simulink model "admire_fcs_lin"  (Simulink 3.00)
settings: Solver=ode4  SolverMode=SingleTasking  StartTime=0.0  StopTime=60  FixedStep=0.008  RelTol=1e-3  AbsTol=1e-6
values from neighbouring files (symbols this model uses):
  x0 = [ max(eyp,zeros(n,1));max(-eyp,zeros(n,1));zeros(2*m,1)]    [LPwrap.m]
undefined symbols (not defined in the file or in its folder): Alt, dalt_err, dMach_err, Mach, u0fcs, y0bare
libraries: simulink3 x22, simulink_extras x8
settings Model: TimeSaveName=tout_split  SaveState=on  StateSaveName=xout_split  OutputSaveName=yout_split  RTWOptions="-aLogVarNameModifier=\"rt_\" -aExtMode=0 -aRollThreshold=5 -aShowEliminatedStatements=1 -aRTWVerbose=1 -aInlineInvariantSignals=1 -aLocalBlockOutputs=1 -aInlineParameters=0"  RTWTemplateMakefile=grt_adm5p3.tmf  LastModifiedBy=lkh  ModifiedComment=nnt -- Mon Jun 05 13:08:11 2000 -- Version 3.42
settings Model: ModifiedHistory=|
  | hkg-- Wed Apr 18 2001: Bug fix: dMach_err and dalt_err are now added to Mach and Alt
  | hkg-- Fri Apr 06 2001: Released with Admire version 3.4d
  | nnt -- Mon Jun 05 13:08:11 2000 -- Version 3.42
  | nnt -- Mon Jun 05 11:01:33 2000 -- Version 3.41
  | nnt -- Mon Jun 05 10:57:40 2000 -- Version 3.40
  | nnt -- Mon Jun 05 10:56:46 2000 -- Version 3.39
  | hkg -- Thu Apr 13 16:38:30 2000 -- Version 3.38
  | Bug fix: all rate limiters were set with the canard parameters, now they get individual settings..
  | hkg -- Thu Apr 13 10:24:31 2000 -- Version 3.37
  | Inserted 3.0 version number in Level 1, changed month to April.
  | hkg -- Tue Apr 11 10:36:55 2000 -- Version 3.36
  | dtz re-connected
  | hkg -- Tue Apr 11 10:28:52 2000 -- Version 3.35
  | Changed the roll force saturation to +-80 N
  | hkg -- Tue Apr 11 09:23:02 2000 -- Version 3.34
  | All signal generators on Level 1 are now set to sine wave
  | hkg -- Mon Apr 10 15:03:16 2000 -- Version 3.33
  | New names for the RL_choice blocks
  | fosimadmin -- Mon Apr 10 13:44:14 2000 -- Version 3.32
  | Hkg actually. Nothing special
  | hkg -- Fri Apr 07 14:32:16 2000 -- Version 3.31
  | A few corrections to the names
  | hkg -- Fri Apr 07 14:16:55 2000 -- Version 3.30
  | Added unique names inside Saab and DASA rate limiters for left elevons, rudder and
  | leading-edge flaps.
  | hkg -- Fri Apr 07 14:04:35 2000 -- Version 3.29
  | Added unique names inside SAAB and DASA rate limiters for canard and right outer and
  | inner elevons.
  | hkg -- Thu Apr 06 17:23:24 2000 -- Version 3.28
  | Inserted unique names for rate limiters and multiport switches in the rate limiter selection blocks.
  | hkg -- Thu Apr 06 16:09:22 2000 -- Version 3.27
  | Disconnected dtz again. Chosen grt_adm5p3.tmf as template makefile. Code generation seems to work.
  | hyd -- Tue Mar 28 15:20:39 2000 -- Version 3.26
  | hyd -- Tue Mar 28 14:28:32 2000 -- Version 3.25
  | hyd -- Tue Mar 28 11:30:24 2000 -- Version 3.24
  | hyd -- Mon Mar 27 15:22:27 2000 -- Version 3.23
  | hyd -- Mon Mar 27 13:42:12 2000 -- Version 3.22
  | hyd -- Mon Mar 27 10:51:54 2000 -- Version 3.21
  | hyd -- Fri Mar 24 13:18:05 2000 -- Version 3.20
  | hyd -- Fri Mar 24 12:50:02 2000 -- Version 3.19
  | hyd -- Fri Mar 24 11:54:23 2000 -- Version 3.18
  | hyd -- Thu Mar 23 15:20:42 2000 -- Version 3.17
  | hyd -- Thu Mar 23 15:17:54 2000 -- Version 3.16
  | hyd -- Wed Mar 22 09:38:49 2000 -- Version 3.15
  | hyd -- Tue Mar 21 14:06:08 2000 -- Version 3.14
  | hyd -- Mon Mar 20 14:42:54 2000 -- Version 3.13
  | hyd -- Wed Mar 15 13:37:48 2000 -- Version 3.12
  | hyd -- Wed Mar 15 12:35:54 2000 -- Version 3.11
  | jnr -- Tue Mar 14 16:36:26 2000 -- Version 3.10
  | jnr -- Tue Mar 14 14:13:39 2000 -- Version 3.9
  | jnr -- Tue Mar 14 14:13:23 2000 -- Version 3.8
  | jnr -- Tue Mar 14 10:09:15 2000 -- Version 3.7
  | jnr -- Tue Mar 14 09:37:34 2000 -- Version 3.6
  | jnr -- Tue Mar 14 09:30:20 2000 -- Version 3.5
  | Add:
  | *proper stick gradients.
  | *correct gains for nz-control according to Åke Hydén.
  | *what transition region between q-control and nz-control is proper??
  | fll -- Fri Mar 03 09:53:48 2000 -- Version 3.4
  | changed name of "dtx" to "dty" (horizontal nozzle deflection)
  | fll -- Thu Mar 02 12:51:23 2000 -- Version 3.3
  | Reducesed the number of integrators to one in the longitudinal controller.
  | fll -- Thu Mar 02 12:30:52 2000 -- Version 3.2
  | Moved the blending function in the Nz and q controller.
  | fll -- Thu Mar 02 10:50:25 2000 -- Version 3.1
  | Changed input blocks to "Signal generator"
  | fll -- Thu Mar 02 10:50:25 2000 -- Version 3.0
  | Version 3.0 is modified according to comments from users

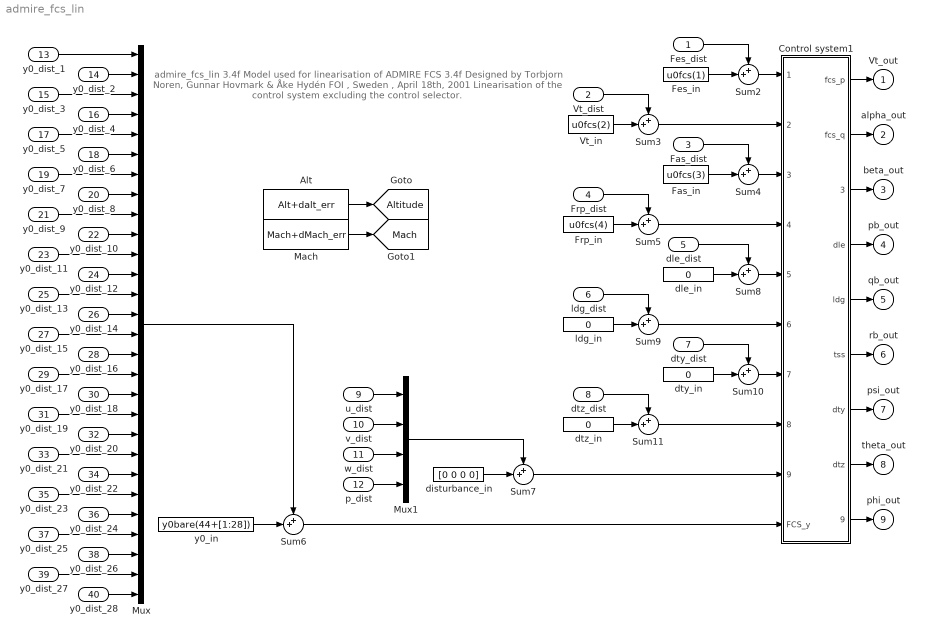
== system admire_fcs_lin ==
  note: admire_fcs_lin 3.4f
      | Model used for linearisation of ADMIRE FCS 3.4f
      | Designed by Torbjorn Noren, Gunnar Hovmark & Åke Hydén
      | FOI , Sweden , April 18th, 2001
      | Linearisation of the control system excluding the
      | control selector.
  Fes_dist : Inport  Port=1  PortWidth=-1  SampleTime=-1  DataType=auto
      settings: SignalType=auto
  Vt_dist : Inport  Port=2  PortWidth=-1  SampleTime=-1  DataType=auto
      settings: SignalType=auto
  Fas_dist : Inport  Port=3  PortWidth=-1  SampleTime=-1  DataType=auto
      settings: SignalType=auto
  Frp_dist : Inport  Port=4  PortWidth=-1  SampleTime=-1  DataType=auto
      settings: SignalType=auto
  dle_dist : Inport  Port=5  PortWidth=-1  SampleTime=-1  DataType=auto
      settings: SignalType=auto
  ldg_dist : Inport  Port=6  PortWidth=-1  SampleTime=-1  DataType=auto
      settings: SignalType=auto
  dty_dist : Inport  Port=7  PortWidth=-1  SampleTime=-1  DataType=auto
      settings: SignalType=auto
  dtz_dist : Inport  Port=8  PortWidth=-1  SampleTime=-1  DataType=auto
      settings: SignalType=auto
  u_dist : Inport  Port=9  PortWidth=-1  SampleTime=-1  DataType=auto
      settings: SignalType=auto
  v_dist : Inport  Port=10  PortWidth=-1  SampleTime=-1  DataType=auto
      settings: SignalType=auto
  w_dist : Inport  Port=11  PortWidth=-1  SampleTime=-1  DataType=auto
      settings: SignalType=auto
  p_dist : Inport  Port=12  PortWidth=-1  SampleTime=-1  DataType=auto
      settings: SignalType=auto
  y0_dist_1 : Inport  Port=13  PortWidth=-1  SampleTime=-1  DataType=auto
      settings: SignalType=auto
  y0_dist_2 : Inport  Port=14  PortWidth=-1  SampleTime=-1  DataType=auto
      settings: SignalType=auto
  y0_dist_3 : Inport  Port=15  PortWidth=-1  SampleTime=-1  DataType=auto
      settings: SignalType=auto
  y0_dist_4 : Inport  Port=16  PortWidth=-1  SampleTime=-1  DataType=auto
      settings: SignalType=auto
  y0_dist_5 : Inport  Port=17  PortWidth=-1  SampleTime=-1  DataType=auto
      settings: SignalType=auto
  y0_dist_6 : Inport  Port=18  PortWidth=-1  SampleTime=-1  DataType=auto
      settings: SignalType=auto
  y0_dist_7 : Inport  Port=19  PortWidth=-1  SampleTime=-1  DataType=auto
      settings: SignalType=auto
  y0_dist_8 : Inport  Port=20  PortWidth=-1  SampleTime=-1  DataType=auto
      settings: SignalType=auto
  y0_dist_9 : Inport  Port=21  PortWidth=-1  SampleTime=-1  DataType=auto
      settings: SignalType=auto
  y0_dist_10 : Inport  Port=22  PortWidth=-1  SampleTime=-1  DataType=auto
      settings: SignalType=auto
  y0_dist_11 : Inport  Port=23  PortWidth=-1  SampleTime=-1  DataType=auto
      settings: SignalType=auto
  y0_dist_12 : Inport  Port=24  PortWidth=-1  SampleTime=-1  DataType=auto
      settings: SignalType=auto
  y0_dist_13 : Inport  Port=25  PortWidth=-1  SampleTime=-1  DataType=auto
      settings: SignalType=auto
  y0_dist_14 : Inport  Port=26  PortWidth=-1  SampleTime=-1  DataType=auto
      settings: SignalType=auto
  y0_dist_15 : Inport  Port=27  PortWidth=-1  SampleTime=-1  DataType=auto
      settings: SignalType=auto
  y0_dist_16 : Inport  Port=28  PortWidth=-1  SampleTime=-1  DataType=auto
      settings: SignalType=auto
  y0_dist_17 : Inport  Port=29  PortWidth=-1  SampleTime=-1  DataType=auto
      settings: SignalType=auto
  y0_dist_18 : Inport  Port=30  PortWidth=-1  SampleTime=-1  DataType=auto
      settings: SignalType=auto
  y0_dist_19 : Inport  Port=31  PortWidth=-1  SampleTime=-1  DataType=auto
      settings: SignalType=auto
  y0_dist_20 : Inport  Port=32  PortWidth=-1  SampleTime=-1  DataType=auto
      settings: SignalType=auto
  y0_dist_21 : Inport  Port=33  PortWidth=-1  SampleTime=-1  DataType=auto
      settings: SignalType=auto
  y0_dist_22 : Inport  Port=34  PortWidth=-1  SampleTime=-1  DataType=auto
      settings: SignalType=auto
  y0_dist_23 : Inport  Port=35  PortWidth=-1  SampleTime=-1  DataType=auto
      settings: SignalType=auto
  y0_dist_24 : Inport  Port=36  PortWidth=-1  SampleTime=-1  DataType=auto
      settings: SignalType=auto
  y0_dist_25 : Inport  Port=37  PortWidth=-1  SampleTime=-1  DataType=auto
      settings: SignalType=auto
  y0_dist_26 : Inport  Port=38  PortWidth=-1  SampleTime=-1  DataType=auto
      settings: SignalType=auto
  y0_dist_27 : Inport  Port=39  PortWidth=-1  SampleTime=-1  DataType=auto
      settings: SignalType=auto
  y0_dist_28 : Inport  Port=40  PortWidth=-1  SampleTime=-1  DataType=auto
      settings: SignalType=auto
  Alt : Constant  Value=Alt+dalt_err
  Control system1 : Subsystem
      mask Display: disp('Control\nSystem')
  Fas_in : Constant  Value=u0fcs(3)
  Fes_in : Constant  Value=u0fcs(1)
  Frp_in : Constant  Value=u0fcs(4)
  Mach : Constant  Value=Mach+dMach_err
  Mux : Mux  Inputs=28
  Mux1 : Mux  Inputs=4
  Sum{2..11} (10 alike) : Sum  Inputs=++|  SaturateOnIntegerOverflow=on
  Vt_in : Constant  Value=u0fcs(2)
  disturbance_in : Constant  Value=[0 0 0 0]
  dle_in : Constant  Value=0
  dty_in : Constant  Value=0
  dtz_in : Constant  Value=0
  ldg_in : Constant  Value=0
  y0_in : Constant  Value=y0bare(44+[1:28])
  Vt_out : Outport  Port=1  InitialOutput=0
  alpha_out : Outport  Port=2  InitialOutput=0
  beta_out : Outport  Port=3  InitialOutput=0
  pb_out : Outport  Port=4  InitialOutput=0
  qb_out : Outport  Port=5  InitialOutput=0
  rb_out : Outport  Port=6  InitialOutput=0
  psi_out : Outport  Port=7  InitialOutput=0
  theta_out : Outport  Port=8  InitialOutput=0
  phi_out : Outport  Port=9  InitialOutput=0
  tag scope: Altitude=global, Mach=global
  wires:
  y0_in/1 -> Sum6/2
  Mux/1 -> Sum6/1
  y0_dist_1/1 -> Mux/1
  y0_dist_2/1 -> Mux/2
  y0_dist_3/1 -> Mux/3
  y0_dist_4/1 -> Mux/4
  y0_dist_5/1 -> Mux/5
  y0_dist_6/1 -> Mux/6
  y0_dist_7/1 -> Mux/7
  y0_dist_8/1 -> Mux/8
  y0_dist_9/1 -> Mux/9
  y0_dist_10/1 -> Mux/10
  y0_dist_11/1 -> Mux/11
  y0_dist_12/1 -> Mux/12
  y0_dist_13/1 -> Mux/13
  y0_dist_14/1 -> Mux/14
  y0_dist_15/1 -> Mux/15
  y0_dist_16/1 -> Mux/16
  y0_dist_17/1 -> Mux/17
  y0_dist_18/1 -> Mux/18
  y0_dist_19/1 -> Mux/19
  y0_dist_20/1 -> Mux/20
  y0_dist_21/1 -> Mux/21
  y0_dist_22/1 -> Mux/22
  y0_dist_23/1 -> Mux/23
  y0_dist_24/1 -> Mux/24
  y0_dist_25/1 -> Mux/25
  y0_dist_26/1 -> Mux/26
  y0_dist_27/1 -> Mux/27
  y0_dist_28/1 -> Mux/28
  Fas_in/1 -> Sum4/2
  Fas_dist/1 -> Sum4/1
  Sum6/1 -> Control system1/10(FCS_y)
  Sum5/1 -> Control system1/4(FCS_Frp)
  Sum4/1 -> Control system1/3(FCS_Fas)
  Sum3/1 -> Control system1/2(FCS_Vt)
  Sum2/1 -> Control system1/1(FCS_Fes)
  dty_in/1 -> Sum10/2
  dty_dist/1 -> Sum10/1
  Sum10/1 -> Control system1/7(FCS_dty)
  Sum9/1 -> Control system1/6(FCS_ldg)
  Sum8/1 -> Control system1/5(FCS_dle)
  Mach/1 -> [Mach]
  Alt/1 -> [Altitude]
  Mux1/1 -> Sum7/1
  disturbance_in/1 -> Sum7/2
  Sum7/1 -> Control system1/9(FCS_dist)
  u_dist/1 -> Mux1/1
  v_dist/1 -> Mux1/2
  w_dist/1 -> Mux1/3
  p_dist/1 -> Mux1/4
  dtz_in/1 -> Sum11/2
  dtz_dist/1 -> Sum11/1
  Sum11/1 -> Control system1/8(FCS_dtz)
  ldg_in/1 -> Sum9/2
  ldg_dist/1 -> Sum9/1
  dle_in/1 -> Sum8/2
  dle_dist/1 -> Sum8/1
  Frp_in/1 -> Sum5/2
  Frp_dist/1 -> Sum5/1
  Vt_in/1 -> Sum3/2
  Vt_dist/1 -> Sum3/1
  Fes_in/1 -> Sum2/2
  Fes_dist/1 -> Sum2/1
  Control system1/1(fcs_p) -> Vt_out/1
  Control system1/2(fcs_q) -> alpha_out/1
  Control system1/3(fcs_beta) -> beta_out/1
  Control system1/4(dle) -> pb_out/1
  Control system1/5(ldg) -> qb_out/1
  Control system1/6(tss) -> rb_out/1
  Control system1/7(dty) -> psi_out/1
  Control system1/8(dtz) -> theta_out/1
  Control system1/9(dis_out) -> phi_out/1

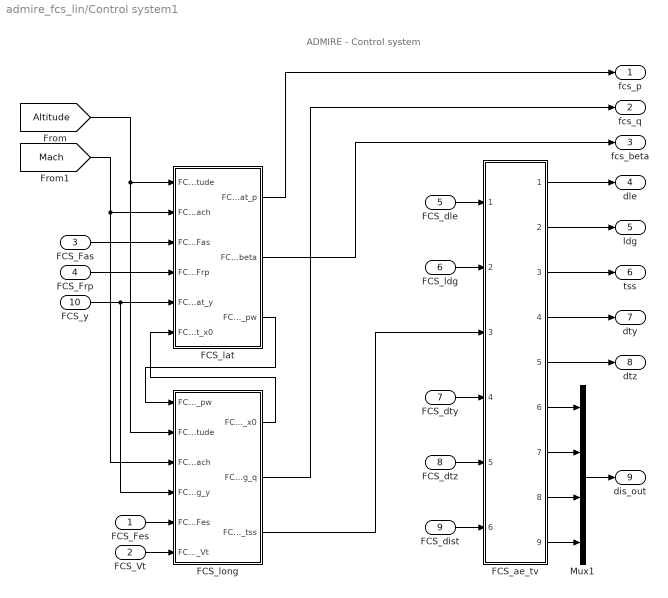
== system admire_fcs_lin/Control system1 ==
  note: ADMIRE - Control system
  FCS_Fes : Inport  Port=1  PortWidth=-1  SampleTime=-1  DataType=auto
      settings: SignalType=auto
  FCS_Vt : Inport  Port=2  PortWidth=-1  SampleTime=-1  DataType=auto
      settings: SignalType=auto
  FCS_Fas : Inport  Port=3  PortWidth=-1  SampleTime=-1  DataType=auto
      settings: SignalType=auto
  FCS_Frp : Inport  Port=4  PortWidth=-1  SampleTime=-1  DataType=auto
      settings: SignalType=auto
  FCS_dle : Inport  Port=5  PortWidth=-1  SampleTime=-1  DataType=auto
      settings: SignalType=auto
  FCS_ldg : Inport  Port=6  PortWidth=-1  SampleTime=-1  DataType=auto
      settings: SignalType=auto
  FCS_dty : Inport  Port=7  PortWidth=-1  SampleTime=-1  DataType=auto
      settings: SignalType=auto
  FCS_dtz : Inport  Port=8  PortWidth=-1  SampleTime=-1  DataType=auto
      settings: SignalType=auto
  FCS_dist : Inport  Port=9  PortWidth=-1  SampleTime=-1  DataType=auto
      settings: SignalType=auto
  FCS_y : Inport  Port=10  PortWidth=-1  SampleTime=-1  DataType=auto
      settings: SignalType=auto
  FCS_ae_tv : Subsystem
      mask Display: disp('Adding\ntrim\nvalues')
  FCS_lat : Subsystem
      mask Display: disp('FCS_lat')
  FCS_long : Subsystem
      mask Display: disp('FCS_long')
  Mux1 : Mux  Inputs=4
  fcs_p : Outport  Port=1
  fcs_q : Outport  Port=2
  fcs_beta : Outport  Port=3
  dle : Outport  Port=4
  ldg : Outport  Port=5
  tss : Outport  Port=6
  dty : Outport  Port=7
  dtz : Outport  Port=8
  dis_out : Outport  Port=9
  wires:
  FCS_long/1(FCS_long_x0) -> FCS_lat/6(FCS_lat_x0)
  FCS_lat/3(FCS_lat_pw) -> FCS_long/1("FCS_long_pw ")
  FCS_Fes/1 -> FCS_long/5(FCS_long_Fes)
  FCS_Vt/1 -> FCS_long/6("FCS_long_Vt ")
  FCS_y/1 -> FCS_lat/5("FCS_lat_y "), FCS_long/4(FCS_long_y)
  FCS_Fas/1 -> FCS_lat/3(FCS_lat_Fas)
  FCS_Frp/1 -> FCS_lat/4(FCS_lat_Frp)
  [Altitude] -> FCS_lat/1("FCS_lat_Altitude "), FCS_long/2("FCS_long_Altitude ")
  [Mach] -> FCS_lat/2("FCS_lat_Mach "), FCS_long/3(FCS_long_Mach)
  FCS_lat/2("FCS_lat_beta ") -> fcs_beta/1
  FCS_long/2(FCS_long_q) -> fcs_q/1
  FCS_ae_tv/1("FCS_ae_tv_dle_out ") -> dle/1
  FCS_ae_tv/2("FCS_ae_tv_ldg_out ") -> ldg/1
  FCS_dle/1 -> FCS_ae_tv/1(FCS_ae_tv_dle)
  FCS_ae_tv/3("FCS_ae_tv_tss_out ") -> tss/1
  FCS_ldg/1 -> FCS_ae_tv/2(FCS_ae_tv_ldg)
  FCS_ae_tv/4(FCS_ae_tv_dty_out) -> dty/1
  FCS_ae_tv/5("FCS_ae_tv_dtz_out ") -> dtz/1
  FCS_dty/1 -> FCS_ae_tv/4(FCS_ae_tv_dty)
  FCS_dtz/1 -> FCS_ae_tv/5(FCS_ae_tv_dtz)
  FCS_dist/1 -> FCS_ae_tv/6(FCS_ae_tv_dist)
  FCS_long/3(FCS_long_tss) -> FCS_ae_tv/3(FCS_ae_tv_tss)
  FCS_lat/1("FCS_lat_p ") -> fcs_p/1
  FCS_ae_tv/9("FCS_ae_tv_p_dist_out ") -> Mux1/4
  FCS_ae_tv/8(FCS_ae_tv_w_dist _out) -> Mux1/3
  FCS_ae_tv/7("FCS_ae_tv_v_dist_out ") -> Mux1/2
  FCS_ae_tv/6("FCS_ae_tv_u_dist_out ") -> Mux1/1
  Mux1/1 -> dis_out/1

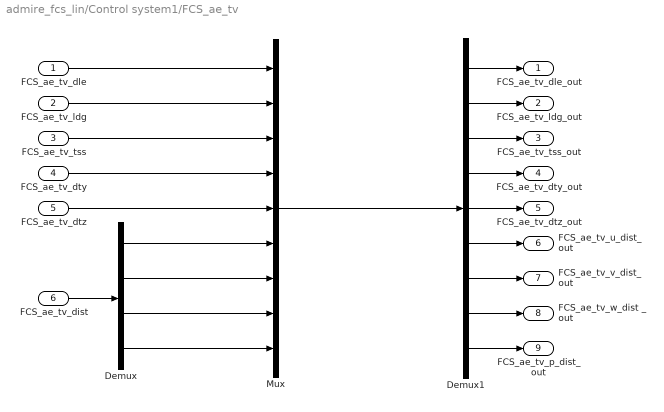
== system admire_fcs_lin/Control system1/FCS_ae_tv ==
  FCS_ae_tv_dle : Inport  Port=1  PortWidth=-1  SampleTime=-1  DataType=auto
      settings: SignalType=auto
  FCS_ae_tv_ldg : Inport  Port=2  PortWidth=-1  SampleTime=-1  DataType=auto
      settings: SignalType=auto
  FCS_ae_tv_tss : Inport  Port=3  PortWidth=-1  SampleTime=-1  DataType=auto
      settings: SignalType=auto
  FCS_ae_tv_dty : Inport  Port=4  PortWidth=-1  SampleTime=-1  DataType=auto
      settings: SignalType=auto
  FCS_ae_tv_dtz : Inport  Port=5  PortWidth=-1  SampleTime=-1  DataType=auto
      settings: SignalType=auto
  FCS_ae_tv_dist : Inport  Port=6  PortWidth=-1  SampleTime=-1  DataType=auto
      settings: SignalType=auto
  Demux : Demux  Outputs=4
  Demux1 : Demux  Outputs=9
  Mux : Mux  Inputs=9
  "FCS_ae_tv_dle_out " : Outport  Port=1
  "FCS_ae_tv_ldg_out " : Outport  Port=2
  "FCS_ae_tv_tss_out " : Outport  Port=3
  FCS_ae_tv_dty_out : Outport  Port=4
  "FCS_ae_tv_dtz_out " : Outport  Port=5
  "FCS_ae_tv_u_dist_out " : Outport  Port=6
  "FCS_ae_tv_v_dist_out " : Outport  Port=7
  FCS_ae_tv_w_dist _out : Outport  Port=8
  "FCS_ae_tv_p_dist_out " : Outport  Port=9
  wires:
  FCS_ae_tv_dist/1 -> Demux/1
  Mux/1 -> Demux1/1
  Demux1/1 -> "FCS_ae_tv_dle_out "/1
  Demux1/4 -> FCS_ae_tv_dty_out/1
  Demux1/5 -> "FCS_ae_tv_dtz_out "/1
  Demux1/6 -> "FCS_ae_tv_u_dist_out "/1
  Demux1/7 -> "FCS_ae_tv_v_dist_out "/1
  Demux1/8 -> FCS_ae_tv_w_dist _out/1
  Demux1/9 -> "FCS_ae_tv_p_dist_out "/1
  FCS_ae_tv_dle/1 -> Mux/1
  FCS_ae_tv_ldg/1 -> Mux/2
  FCS_ae_tv_tss/1 -> Mux/3
  FCS_ae_tv_dty/1 -> Mux/4
  FCS_ae_tv_dtz/1 -> Mux/5
  Demux/1 -> Mux/6
  Demux/2 -> Mux/7
  Demux/3 -> Mux/8
  Demux/4 -> Mux/9
  Demux1/2 -> "FCS_ae_tv_ldg_out "/1
  Demux1/3 -> "FCS_ae_tv_tss_out "/1

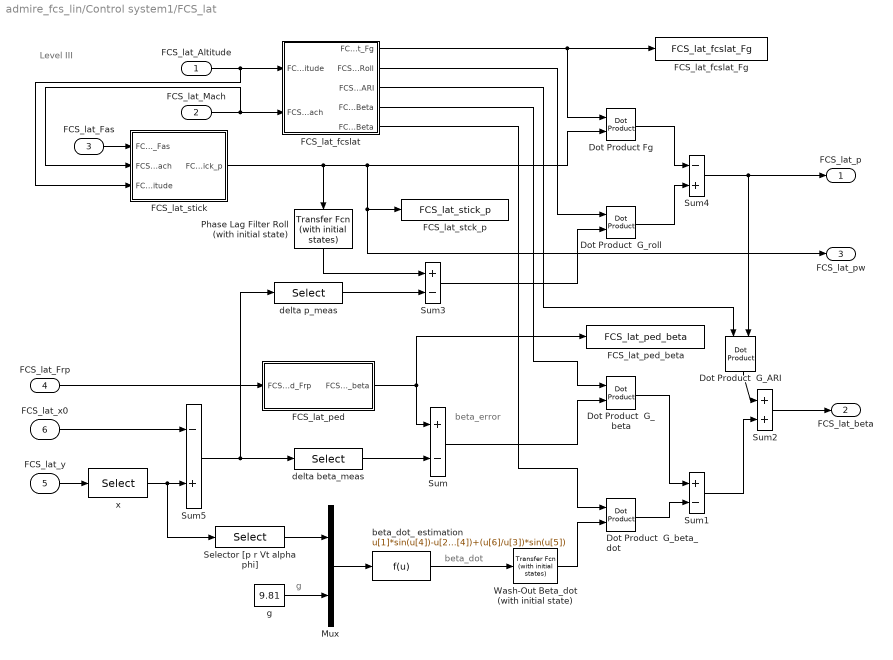
== system admire_fcs_lin/Control system1/FCS_lat ==
  note: g
  note: beta_dot
  note: beta_error
  note: Level III
  "FCS_lat_Altitude " : Inport  Port=1  PortWidth=-1  SampleTime=-1  DataType=auto
      settings: SignalType=auto
  "FCS_lat_Mach " : Inport  Port=2  PortWidth=-1  SampleTime=-1  DataType=auto
      settings: SignalType=auto
  FCS_lat_Fas : Inport  Port=3  PortWidth=-1  SampleTime=-1  DataType=auto
      settings: SignalType=auto
  FCS_lat_Frp : Inport  Port=4  PortWidth=-1  SampleTime=-1  DataType=auto
      settings: SignalType=auto
  "FCS_lat_y " : Inport  Port=5  PortWidth=-1  SampleTime=-1  DataType=auto
      settings: SignalType=auto
  FCS_lat_x0 : Inport  Port=6  PortWidth=-1  SampleTime=-1  DataType=auto
      settings: SignalType=auto
  "  x" : Selector  Elements=[1:12]  InputPortWidth=28
  Dot Product Fg : simulink3/Math/Dot Product
  Dot Product  G_ARI : simulink3/Math/Dot Product  Orientation=down
  Dot Product  G_beta : simulink3/Math/Dot Product
  Dot Product  G_beta_dot : simulink3/Math/Dot Product
  Dot Product  G_roll : simulink3/Math/Dot Product
  FCS_lat_fcslat : Subsystem
      mask Display: disp('Calc of lateral\namplfication\n factors')
  FCS_lat_fcslat_Fg : ToWorkspace  VariableName=FCS_lat_fcslat_Fg  SampleTime=-1  SaveFormat=Matrix
  FCS_lat_ped : Subsystem
      mask Display: disp('FCS lateral pedal\nforce N to beta rad')
  FCS_lat_ped_beta : ToWorkspace  VariableName=FCS_lat_ped_beta  SampleTime=-1  SaveFormat=Matrix
  FCS_lat_stck_p : ToWorkspace  VariableName=FCS_lat_stick_p  SampleTime=-1  SaveFormat=Matrix
  FCS_lat_stick : Subsystem
      mask Display: disp('FCS lateral stick\ngradient\n N to rad/s')
  Mux : Mux  Inputs=2
      settings: DisplayOption=none
  Phase Lag Filter Roll (with initial state) : simulink_extras/Additional Linear/Transfer Fcn (with initial states)  Orientation=down  N=[0 1]  D="[0.25  1]"  X0=x0(39)
  Selector [p r Vt alpha phi] : Selector  Elements=[4 6 1 2 9]  InputPortWidth=12
  Sum : Sum  Inputs=+-  SaturateOnIntegerOverflow=on
  Sum1 : Sum  Inputs=+-  SaturateOnIntegerOverflow=on
  Sum2 : Sum  Inputs=++  SaturateOnIntegerOverflow=on
  Sum3 : Sum  Inputs=+-  SaturateOnIntegerOverflow=on
  Sum4 : Sum  Inputs=-+  SaturateOnIntegerOverflow=on
  Sum5 : Sum  Inputs=-+  SaturateOnIntegerOverflow=on
  Wash-Out Beta_dot (with initial state) : simulink_extras/Additional Linear/Transfer Fcn (with initial states)  N=[5 0]  D="[5  1]"  X0=x0(40)
  beta_dot_ estimation : Fcn  Expr=u[1]*sin(u[4])-u[2]*cos(u[4])+(u[6]/u[3])*sin(u[5])
  delta beta_meas : Selector  Elements=3  InputPortWidth=12
  delta p_meas : Selector  Elements=4  InputPortWidth=12
  g : Constant  Value=9.81
  "FCS_lat_p " : Outport  Port=1  InitialOutput=0
  "FCS_lat_beta " : Outport  Port=2  InitialOutput=0
  FCS_lat_pw : Outport  Port=3  InitialOutput=0
  wires:
  FCS_lat_Fas/1 -> FCS_lat_stick/1("FCS_lat_stick_Fas ")
  Phase Lag Filter Roll (with initial state)/1 -> Sum3/1
  delta p_meas/1 -> Sum3/2
  Mux/1 -> beta_dot_ estimation/1
  Selector [p r Vt alpha phi]/1 -> Mux/1
  g/1 -> Mux/2
  beta_dot_ estimation/1 -> Wash-Out Beta_dot (with initial state)/1
  Sum3/1 -> Dot Product  G_roll/2
  Dot Product  G_roll/1 -> Sum4/2
  Dot Product Fg/1 -> Sum4/1
  Wash-Out Beta_dot (with initial state)/1 -> Dot Product  G_beta_dot/2
  Dot Product  G_beta/1 -> Sum1/1
  Dot Product  G_beta_dot/1 -> Sum1/2
  Sum4/1 -> Dot Product  G_ARI/2, "FCS_lat_p "/1
  Dot Product  G_ARI/1 -> Sum2/1
  Sum2/1 -> "FCS_lat_beta "/1
  Sum1/1 -> Sum2/2
  FCS_lat_stick/1(FCS_lat_stick_p) -> Phase Lag Filter Roll (with initial state)/1, Dot Product Fg/2, FCS_lat_pw/1, FCS_lat_stck_p/1
  FCS_lat_fcslat/2(FCS_lat_fcslat_GRoll) -> Dot Product  G_roll/1
  FCS_lat_fcslat/3(FCS_lat_fcslat_GARI) -> Dot Product  G_ARI/1
  FCS_lat_fcslat/4(FCS_lat_fcslat_GBeta) -> Dot Product  G_beta/1
  FCS_lat_fcslat/5(FCS_lat_fcslat_dGBeta) -> Dot Product  G_beta_dot/1
  delta beta_meas/1 -> Sum/2
  Sum/1 -> Dot Product  G_beta/2
  FCS_lat_Frp/1 -> FCS_lat_ped/1(FCS_lat_ped_Frp)
  FCS_lat_ped/1(FCS_lat_ped_beta) -> Sum/1, FCS_lat_ped_beta/1
  "FCS_lat_Altitude "/1 -> FCS_lat_fcslat/1(FCS_lat_fcslat_Altitude), FCS_lat_stick/3("FCS_lat_stick_Altitude ")
  "FCS_lat_Mach "/1 -> FCS_lat_stick/2("FCS_lat_stick_Mach "), FCS_lat_fcslat/2(FCS_lat_fcslat_Mach)
  "FCS_lat_y "/1 -> "  x"/1
  FCS_lat_x0/1 -> Sum5/1
  "  x"/1 -> Sum5/2, Selector [p r Vt alpha phi]/1
  Sum5/1 -> delta beta_meas/1, delta p_meas/1
  FCS_lat_fcslat/1(FCS_lat_fcslat_Fg) -> Dot Product Fg/1, FCS_lat_fcslat_Fg/1

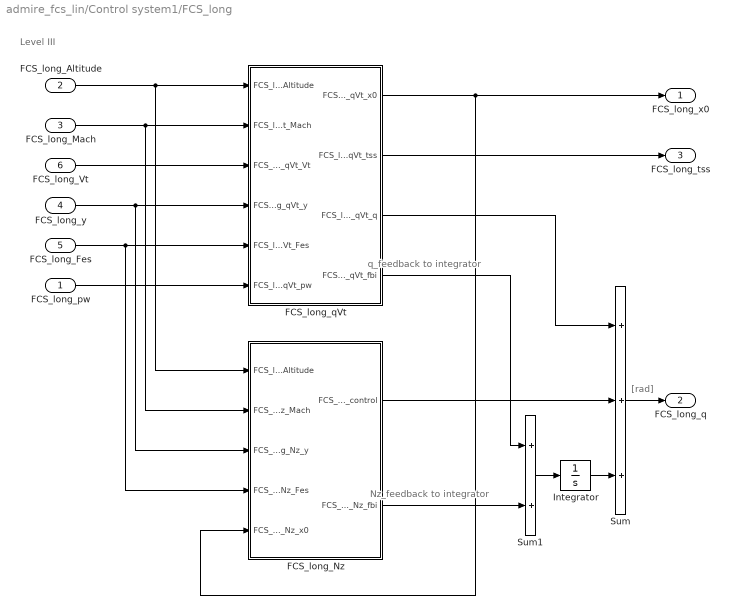
== system admire_fcs_lin/Control system1/FCS_long ==
  note: Level III
  note: q_feedback
      | to integrator
  note: Nz_feedback
      | to integrator
  note: [rad]
  "FCS_long_pw " : Inport  Port=1  PortWidth=-1  SampleTime=-1  DataType=auto
      settings: SignalType=auto
  "FCS_long_Altitude " : Inport  Port=2  PortWidth=-1  SampleTime=-1  DataType=auto
      settings: SignalType=auto
  FCS_long_Mach : Inport  Port=3  PortWidth=-1  SampleTime=-1  DataType=auto
      settings: SignalType=auto
  FCS_long_y : Inport  Port=4  PortWidth=-1  SampleTime=-1  DataType=auto
      settings: SignalType=auto
  FCS_long_Fes : Inport  Port=5  PortWidth=-1  SampleTime=-1  DataType=auto
      settings: SignalType=auto
  "FCS_long_Vt " : Inport  Port=6  PortWidth=-1  SampleTime=-1  DataType=auto
      settings: SignalType=auto
  FCS_long_Nz : Subsystem
      mask Display: disp('FCS_long_Nz')
  FCS_long_qVt : Subsystem
      mask Display: disp('FCS_long_qVt')
  Integrator : Integrator  ExternalReset=none  InitialConditionSource=internal  InitialCondition=0  LimitOutput=off  UpperSaturationLimit=inf  LowerSaturationLimit=-inf  ShowSaturationPort=off  ShowStatePort=off  AbsoluteTolerance=auto
  Sum : Sum  Inputs=+++  SaturateOnIntegerOverflow=on
  Sum1 : Sum  Inputs=++  SaturateOnIntegerOverflow=on
  FCS_long_x0 : Outport  Port=1  InitialOutput=0
  FCS_long_q : Outport  Port=2  InitialOutput=0
  FCS_long_tss : Outport  Port=3  InitialOutput=0
  wires:
  "FCS_long_Vt "/1 -> FCS_long_qVt/3(FCS_long_qVt_Vt)
  FCS_long_Mach/1 -> FCS_long_qVt/2(FCS_long_qVt_Mach), FCS_long_Nz/2("FCS_long_Nz_Mach ")
  FCS_long_y/1 -> FCS_long_qVt/4(FCS_long_qVt_y), FCS_long_Nz/3(FCS_long_Nz_y)
  FCS_long_qVt/1(FCS_long_qVt_x0) -> FCS_long_x0/1, FCS_long_Nz/5(FCS_long_Nz_x0)
  FCS_long_Fes/1 -> FCS_long_qVt/5(FCS_long_qVt_Fes), FCS_long_Nz/4(FCS_long_Nz_Fes)
  "FCS_long_pw "/1 -> FCS_long_qVt/6("FCS_long_qVt_pw ")
  FCS_long_qVt/2(FCS_long_qVt_tss) -> FCS_long_tss/1
  FCS_long_qVt/3(FCS_long_qVt_q) -> Sum/1
  FCS_long_Nz/1(FCS_long_Nz_control) -> Sum/2
  FCS_long_qVt/4(FCS_long_qVt_fbi) -> Sum1/1
  FCS_long_Nz/2(FCS_long_Nz_fbi) -> Sum1/2
  Integrator/1 -> Sum/3
  "FCS_long_Altitude "/1 -> FCS_long_qVt/1(FCS_long_qVt_Altitude), FCS_long_Nz/1("FCS_long_Nz_Altitude ")
  Sum/1 -> FCS_long_q/1
  Sum1/1 -> Integrator/1

== system admire_fcs_lin/Control system1/FCS_lat/FCS_lat_fcslat ==
  note: Level IV
  note: S-function
  FCS_lat_fcslat_Altitude : Inport  Port=1  PortWidth=-1  SampleTime=-1  DataType=auto
      settings: SignalType=auto
  FCS_lat_fcslat_Mach : Inport  Port=2  PortWidth=-1  SampleTime=-1  DataType=auto
      settings: SignalType=auto
  S-Function : S-Function  FunctionName=fcslateral  PortCounts=[]  SFunctionModules=''
  FCS_lat_fcslat_Fg : Outport  Port=1
  FCS_lat_fcslat_GRoll : Outport  Port=2
  FCS_lat_fcslat_GARI : Outport  Port=3
  FCS_lat_fcslat_GBeta : Outport  Port=4
  FCS_lat_fcslat_dGBeta : Outport  Port=5
  wires:
  FCS_lat_fcslat_Altitude/1 -> S-Function/1
  FCS_lat_fcslat_Mach/1 -> S-Function/2
  S-Function/1 -> FCS_lat_fcslat_Fg/1
  S-Function/2 -> FCS_lat_fcslat_GBeta/1
  S-Function/3 -> FCS_lat_fcslat_dGBeta/1
  S-Function/4 -> FCS_lat_fcslat_GARI/1
  S-Function/5 -> FCS_lat_fcslat_GRoll/1

== system admire_fcs_lin/Control system1/FCS_lat/FCS_lat_ped ==
  note: Level IV
  FCS_lat_ped_Frp : Inport  Port=1  PortWidth=-1  SampleTime=-1  DataType=auto
      settings: SignalType=auto
  Degrees to Radians : simulink_extras/Transformations/Degrees to Radians
  Look-Up Table Frp gradient : Lookup  InputValues=[-200 0 200]  OutputValues=[5 0 -5]
  Saturation : Saturate  UpperLimit=200  LowerLimit=-200
  FCS_lat_ped_beta : Outport  Port=1
  wires:
  Saturation/1 -> Look-Up Table Frp gradient/1
  FCS_lat_ped_Frp/1 -> Saturation/1
  Degrees to Radians/1 -> FCS_lat_ped_beta/1
  Look-Up Table Frp gradient/1 -> Degrees to Radians/1

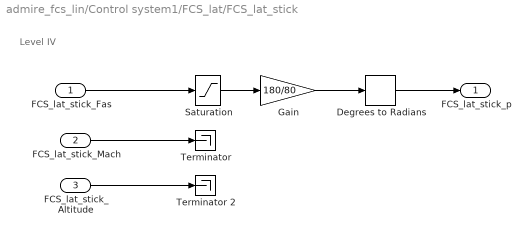
== system admire_fcs_lin/Control system1/FCS_lat/FCS_lat_stick ==
  note: Level IV
  "FCS_lat_stick_Fas " : Inport  Port=1  PortWidth=-1  SampleTime=-1  DataType=auto
      settings: SignalType=auto
  "FCS_lat_stick_Mach " : Inport  Port=2  PortWidth=-1  SampleTime=-1  DataType=auto
      settings: SignalType=auto
  "FCS_lat_stick_Altitude " : Inport  Port=3  PortWidth=-1  SampleTime=-1  DataType=auto
      settings: SignalType=auto
  Degrees to Radians : simulink_extras/Transformations/Degrees to Radians
  Gain : Gain  Gain=180/80  SaturateOnIntegerOverflow=on
  Saturation : Saturate  UpperLimit=80  LowerLimit=-80
  Terminator : Terminator
  Terminator 2 : Terminator
  FCS_lat_stick_p : Outport  Port=1
  wires:
  "FCS_lat_stick_Fas "/1 -> Saturation/1
  Degrees to Radians/1 -> FCS_lat_stick_p/1
  Saturation/1 -> Gain/1
  Gain/1 -> Degrees to Radians/1
  "FCS_lat_stick_Mach "/1 -> Terminator/1
  "FCS_lat_stick_Altitude "/1 -> Terminator 2/1

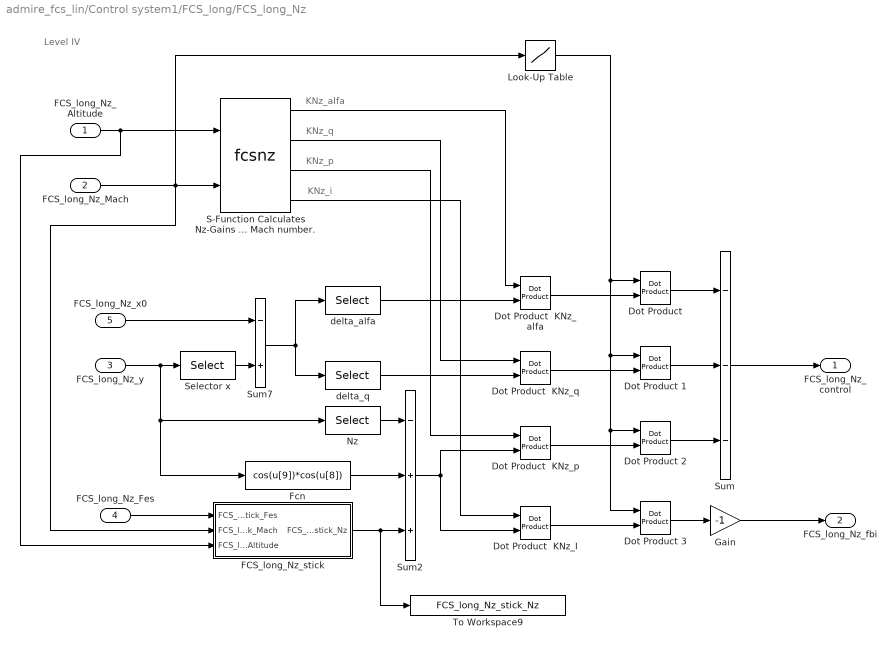
== system admire_fcs_lin/Control system1/FCS_long/FCS_long_Nz ==
  note: KNz_alfa
  note: KNz_q
  note: KNz_p
  note: KNz_i
  note: Level IV
  "FCS_long_Nz_Altitude " : Inport  Port=1  PortWidth=-1  SampleTime=-1  DataType=auto
      settings: SignalType=auto
  "FCS_long_Nz_Mach " : Inport  Port=2  PortWidth=-1  SampleTime=-1  DataType=auto
      settings: SignalType=auto
  FCS_long_Nz_y : Inport  Port=3  PortWidth=-1  SampleTime=-1  DataType=auto
      settings: SignalType=auto
  FCS_long_Nz_Fes : Inport  Port=4  PortWidth=-1  SampleTime=-1  DataType=auto
      settings: SignalType=auto
  FCS_long_Nz_x0 : Inport  Port=5  PortWidth=-1  SampleTime=-1  DataType=auto
      settings: SignalType=auto
  Dot Product {,1..3} (4 alike) : simulink3/Math/Dot Product
  Dot Product  KNz_I : simulink3/Math/Dot Product
  Dot Product  KNz_alfa : simulink3/Math/Dot Product
  Dot Product  KNz_p : simulink3/Math/Dot Product
  Dot Product  KNz_q : simulink3/Math/Dot Product
  FCS_long_Nz_stick : Subsystem
      mask Display: disp('FCS_long_Nz_stick')
  Fcn : Fcn  Expr=cos(u[9])*cos(u[8])
  Gain : Gain  Gain=-1  SaturateOnIntegerOverflow=on
  Look-Up Table : Lookup  InputValues=[0 0.58 0.62 2.5]  OutputValues=[0 0 1 1]
  Nz : Selector  Elements=19  InputPortWidth=28
  S-Function Calculates Nz-Gains as a function of altitude and Mach number. : S-Function  FunctionName=fcsnz  PortCounts=[]  SFunctionModules=''
  Selector x : Selector  Elements=[1:12]  InputPortWidth=28
  Sum : Sum  Inputs=---  SaturateOnIntegerOverflow=on
  Sum2 : Sum  Inputs=-++  SaturateOnIntegerOverflow=on
  Sum7 : Sum  Inputs=-+  SaturateOnIntegerOverflow=on
  To Workspace9 : ToWorkspace  VariableName=FCS_long_Nz_stick_Nz  SampleTime=-1  SaveFormat=Matrix
  delta_alfa : Selector  Elements=2  InputPortWidth=12
  delta_q : Selector  Elements=5  InputPortWidth=12
  FCS_long_Nz_control : Outport  Port=1
  FCS_long_Nz_fbi : Outport  Port=2
  wires:
  Nz/1 -> Sum2/1
  FCS_long_Nz_Fes/1 -> FCS_long_Nz_stick/1("FCS_long_Nz_stick_Fes ")
  Selector x/1 -> Sum7/2
  FCS_long_Nz_x0/1 -> Sum7/1
  Sum7/1 -> delta_alfa/1, delta_q/1
  FCS_long_Nz_y/1 -> Selector x/1, Nz/1, Fcn/1
  "FCS_long_Nz_Mach "/1 -> S-Function Calculates Nz-Gains as a function of altitude and Mach number./2, Look-Up Table/1, FCS_long_Nz_stick/2(FCS_long_Nz_stick_Mach)
  Sum2/1 -> Dot Product  KNz_p/2, Dot Product  KNz_I/2
  S-Function Calculates Nz-Gains as a function of altitude and Mach number./4 -> Dot Product  KNz_I/1
  delta_alfa/1 -> Dot Product  KNz_alfa/2
  delta_q/1 -> Dot Product  KNz_q/2
  S-Function Calculates Nz-Gains as a function of altitude and Mach number./3 -> Dot Product  KNz_p/1
  S-Function Calculates Nz-Gains as a function of altitude and Mach number./2 -> Dot Product  KNz_q/1
  S-Function Calculates Nz-Gains as a function of altitude and Mach number./1 -> Dot Product  KNz_alfa/1
  "Dot Product "/1 -> Sum/1
  Dot Product  KNz_alfa/1 -> "Dot Product "/2
  Dot Product 1/1 -> Sum/2
  Dot Product  KNz_q/1 -> Dot Product 1/2
  Look-Up Table/1 -> "Dot Product "/1, Dot Product 1/1, Dot Product 2/1, Dot Product 3/1
  Dot Product 2/1 -> Sum/3
  Dot Product  KNz_p/1 -> Dot Product 2/2
  Dot Product  KNz_I/1 -> Dot Product 3/2
  Sum/1 -> FCS_long_Nz_control/1
  Gain/1 -> FCS_long_Nz_fbi/1
  Dot Product 3/1 -> Gain/1
  "FCS_long_Nz_Altitude "/1 -> S-Function Calculates Nz-Gains as a function of altitude and Mach number./1, FCS_long_Nz_stick/3("FCS_long_Nz_stick_Altitude ")
  FCS_long_Nz_stick/1(FCS_long_Nz_stick_Nz) -> To Workspace9/1, Sum2/3
  Fcn/1 -> Sum2/2

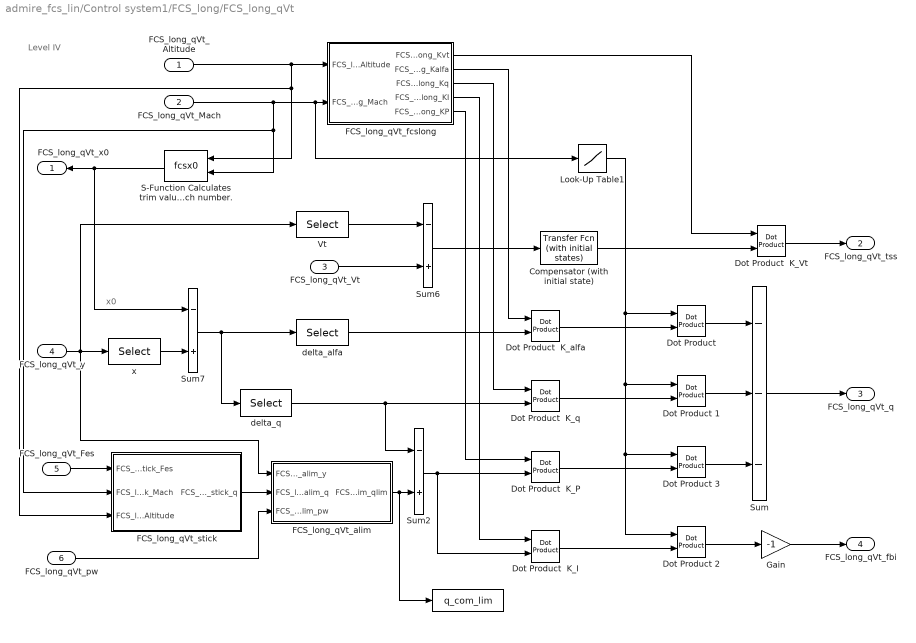
== system admire_fcs_lin/Control system1/FCS_long/FCS_long_qVt ==
  note: x0
  note: Level IV
  FCS_long_qVt_Altitude : Inport  Port=1  PortWidth=-1  SampleTime=-1  DataType=auto
      settings: SignalType=auto
  FCS_long_qVt_Mach : Inport  Port=2  PortWidth=-1  SampleTime=-1  DataType=auto
      settings: SignalType=auto
  FCS_long_qVt_Vt : Inport  Port=3  PortWidth=-1  SampleTime=-1  DataType=auto
      settings: SignalType=auto
  FCS_long_qVt_y : Inport  Port=4  PortWidth=-1  SampleTime=-1  DataType=auto
      settings: SignalType=auto
  FCS_long_qVt_Fes : Inport  Port=5  PortWidth=-1  SampleTime=-1  DataType=auto
      settings: SignalType=auto
  "FCS_long_qVt_pw " : Inport  Port=6  PortWidth=-1  SampleTime=-1  DataType=auto
      settings: SignalType=auto
  " " : ToWorkspace  VariableName=q_com_lim  SampleTime=-1  SaveFormat=Matrix
  Compensator (with initial state) : simulink_extras/Additional Linear/Transfer Fcn (with initial states)  N=[15 10]  D="[1  10]"  X0=x0(41)
  Dot Product {,1..3} (4 alike) : simulink3/Math/Dot Product
  Dot Product  K_I : simulink3/Math/Dot Product
  Dot Product  K_P : simulink3/Math/Dot Product
  Dot Product  K_Vt : simulink3/Math/Dot Product
  Dot Product  K_alfa : simulink3/Math/Dot Product
  Dot Product  K_q : simulink3/Math/Dot Product
  FCS_long_qVt_alim : Subsystem
      mask Display: disp('FCS_long_qVt_alim')
  FCS_long_qVt_fcslong : Subsystem
      mask Display: disp('FCS_long_qVt_fcslong')
  FCS_long_qVt_stick : Subsystem
      mask Display: disp('FCS_long_qVt_stick')
  Gain : Gain  Gain=-1  SaturateOnIntegerOverflow=on
  Look-Up Table1 : Lookup  InputValues=[0 0.58 0.62 2.5]  OutputValues=[1 1 0 0]
  "S-Function Calculates trim values, x0, as a function of altitude and Mach number." : S-Function  Orientation=left  FunctionName=fcsx0  PortCounts=[]  SFunctionModules=''
  Sum : Sum  Inputs=---  SaturateOnIntegerOverflow=on
  Sum2 : Sum  Inputs=-+  SaturateOnIntegerOverflow=on
  Sum6 : Sum  Inputs=-+  SaturateOnIntegerOverflow=on
  Sum7 : Sum  Inputs=-+  SaturateOnIntegerOverflow=on
  Vt : Selector  Elements=1  InputPortWidth=28
  delta_alfa : Selector  Elements=2  InputPortWidth=12
  delta_q : Selector  Elements=5  InputPortWidth=12
  x : Selector  Elements=[1:12]  InputPortWidth=28
  FCS_long_qVt_x0 : Outport  Orientation=left  Port=1
  FCS_long_qVt_tss : Outport  Port=2
  FCS_long_qVt_q : Outport  Port=3
  FCS_long_qVt_fbi : Outport  Port=4
  wires:
  FCS_long_qVt_fcslong/4(FCS_long_qVt_fcslong_KI) -> Dot Product  K_I/1
  FCS_long_qVt_fcslong/5(FCS_long_qVt_fcslong_KP) -> Dot Product  K_P/1
  FCS_long_qVt_Altitude/1 -> FCS_long_qVt_fcslong/1(FCS_long_qVt_fcslong_Altitude), "S-Function Calculates trim values, x0, as a function of altitude and Mach number."/1, FCS_long_qVt_stick/3("FCS_long_qVt_stick_Altitude ")
  FCS_long_qVt_Mach/1 -> FCS_long_qVt_fcslong/2(FCS_long_qVt_fcslong_Mach), Look-Up Table1/1, "S-Function Calculates trim values, x0, as a function of altitude and Mach number."/2, FCS_long_qVt_stick/2("FCS_long_qVt_stick_Mach ")
  delta_alfa/1 -> Dot Product  K_alfa/2
  x/1 -> Sum7/2
  Sum7/1 -> delta_alfa/1, delta_q/1
  delta_q/1 -> Dot Product  K_q/2, Sum2/1
  FCS_long_qVt_y/1 -> x/1, Vt/1, FCS_long_qVt_alim/1(FCS_long_qVt_alim_y)
  "S-Function Calculates trim values, x0, as a function of altitude and Mach number."/1 -> Sum7/1, FCS_long_qVt_x0/1
  FCS_long_qVt_Fes/1 -> FCS_long_qVt_stick/1("FCS_long_qVt_stick_Fes ")
  FCS_long_qVt_alim/1(FCS_long_qVt_alim_qlim) -> Sum2/2, " "/1
  FCS_long_qVt_stick/1("FCS_long_qVt_stick_q ") -> FCS_long_qVt_alim/2("FCS_long_qVt_alim_q ")
  "FCS_long_qVt_pw "/1 -> FCS_long_qVt_alim/3(FCS_long_qVt_alim_pw)
  Compensator (with initial state)/1 -> Dot Product  K_Vt/2
  Dot Product  K_Vt/1 -> FCS_long_qVt_tss/1
  FCS_long_qVt_fcslong/1(FCS_long_qVt_fcslong_Kvt) -> Dot Product  K_Vt/1
  Sum2/1 -> Dot Product  K_P/2, Dot Product  K_I/2
  Dot Product  K_P/1 -> Dot Product 3/2
  Dot Product  K_I/1 -> Dot Product 2/2
  Sum/1 -> FCS_long_qVt_q/1
  Dot Product  K_q/1 -> Dot Product 1/2
  Dot Product 1/1 -> Sum/2
  "Dot Product "/1 -> Sum/1
  Dot Product  K_alfa/1 -> "Dot Product "/2
  Look-Up Table1/1 -> "Dot Product "/1, Dot Product 1/1, Dot Product 2/1, Dot Product 3/1
  Vt/1 -> Sum6/1
  FCS_long_qVt_Vt/1 -> Sum6/2
  Sum6/1 -> Compensator (with initial state)/1
  Dot Product 3/1 -> Sum/3
  Gain/1 -> FCS_long_qVt_fbi/1
  Dot Product 2/1 -> Gain/1
  FCS_long_qVt_fcslong/3(FCS_long_qVt_fcslong_Kq) -> Dot Product  K_q/1
  FCS_long_qVt_fcslong/2(FCS_long_qVt_fcslong_Kalfa) -> Dot Product  K_alfa/1

== system admire_fcs_lin/Control system1/FCS_long/FCS_long_Nz/FCS_long_Nz_stick ==
  note: Level V
  "FCS_long_Nz_stick_Fes " : Inport  Port=1  PortWidth=-1  SampleTime=-1  DataType=auto
      settings: SignalType=auto
  FCS_long_Nz_stick_Mach : Inport  Port=2  PortWidth=-1  SampleTime=-1  DataType=auto
      settings: SignalType=auto
  "FCS_long_Nz_stick_Altitude " : Inport  Port=3  PortWidth=-1  SampleTime=-1  DataType=auto
      settings: SignalType=auto
  Gain : Gain  Gain=8/80  SaturateOnIntegerOverflow=on
  Saturation [-40,+80]   [Newton] : Saturate  UpperLimit=80  LowerLimit=-40
  Terminator : Terminator
  Terminator 2 : Terminator
  FCS_long_Nz_stick_Nz : Outport  Port=1
  wires:
  "FCS_long_Nz_stick_Fes "/1 -> Saturation [-40,+80]   [Newton]/1
  Saturation [-40,+80]   [Newton]/1 -> Gain/1
  Gain/1 -> FCS_long_Nz_stick_Nz/1
  "FCS_long_Nz_stick_Altitude "/1 -> Terminator 2/1
  FCS_long_Nz_stick_Mach/1 -> Terminator/1

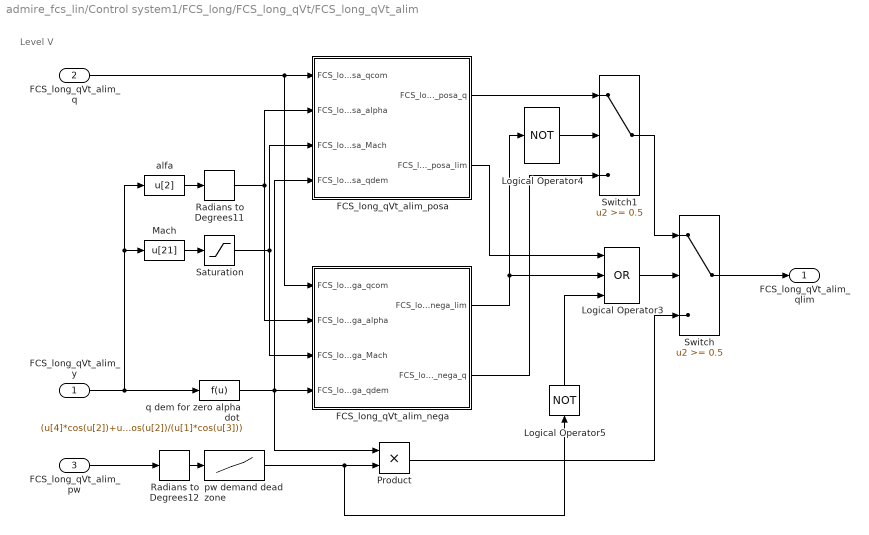
== system admire_fcs_lin/Control system1/FCS_long/FCS_long_qVt/FCS_long_qVt_alim ==
  note: Level V
  FCS_long_qVt_alim_y : Inport  Port=1  PortWidth=-1  SampleTime=-1  DataType=auto
      settings: SignalType=auto
  "FCS_long_qVt_alim_q " : Inport  Port=2  PortWidth=-1  SampleTime=-1  DataType=auto
      settings: SignalType=auto
  FCS_long_qVt_alim_pw : Inport  Port=3  PortWidth=-1  SampleTime=-1  DataType=auto
      settings: SignalType=auto
  FCS_long_qVt_alim_nega : Subsystem
      mask Display: disp('FCS_long_qVt_alim\nnegative alpha')
  FCS_long_qVt_alim_posa : Subsystem
      mask Display: disp('FCS_long_qVt_alim\npositive alpha')
  Logical Operator3 : Logic  Operator=OR  Inputs=3
  Logical Operator4 : Logic  Operator=NOT  Inputs=1
  Logical Operator5 : Logic  Orientation=up  Operator=NOT  Inputs=1
  Mach : Fcn  Expr=u[21]
  Product : Product  Inputs=2  SaturateOnIntegerOverflow=on
  Radians to Degrees11 : simulink_extras/Transformations/Radians to Degrees
  Radians to Degrees12 : simulink_extras/Transformations/Radians to Degrees
  Saturation : Saturate  UpperLimit=2.5  LowerLimit=0
  Switch : Switch  Threshold=0.5
  Switch1 : Switch  Threshold=0.5
  alfa : Fcn  Expr=u[2]
  pw demand dead zone : Lookup  InputValues=[-180 -10 -8 8 10 180]  OutputValues=[0 0 0 0 0 0]
  "q dem for zero alpha dot " : Fcn  Expr=(u[4]*cos(u[2])+u[6]*sin(u[2]))*tan(u[3])+(u[19]-cos(u[8])*cos(u[9]))*9.80665*cos(u[2])/(u[1]*cos(u[3]))
  FCS_long_qVt_alim_qlim : Outport  Port=1
  wires:
  Logical Operator3/1 -> Switch/2
  Switch1/1 -> Switch/1
  alfa/1 -> Radians to Degrees11/1
  Mach/1 -> Saturation/1
  Radians to Degrees11/1 -> FCS_long_qVt_alim_posa/2("FCS_long_qVt_alim_posa_alpha "), FCS_long_qVt_alim_nega/2("FCS_long_qVt_alim_nega_alpha ")
  Saturation/1 -> FCS_long_qVt_alim_posa/3("FCS_long_qVt_alim_posa_Mach "), FCS_long_qVt_alim_nega/3("FCS_long_qVt_alim_nega_Mach ")
  FCS_long_qVt_alim_y/1 -> "q dem for zero alpha dot "/1, Mach/1, alfa/1
  "q dem for zero alpha dot "/1 -> FCS_long_qVt_alim_nega/4("FCS_long_qVt_alim_nega_qdem "), FCS_long_qVt_alim_posa/4("FCS_long_qVt_alim_posa_qdem "), Product/1
  "FCS_long_qVt_alim_q "/1 -> FCS_long_qVt_alim_posa/1("FCS_long_qVt_alim_posa_qcom "), FCS_long_qVt_alim_nega/1("FCS_long_qVt_alim_nega_qcom ")
  FCS_long_qVt_alim_nega/2("FCS_long_qVt_alim_nega_q ") -> Switch1/3
  FCS_long_qVt_alim_posa/1(FCS_long_qVt_alim_posa_q) -> Switch1/1
  Logical Operator4/1 -> Switch1/2
  FCS_long_qVt_alim_nega/1(FCS_long_qVt_alim_nega_lim) -> Logical Operator4/1, Logical Operator3/2
  FCS_long_qVt_alim_posa/2(FCS_long_qVt_alim_posa_lim) -> Logical Operator3/1
  Switch/1 -> FCS_long_qVt_alim_qlim/1
  Radians to Degrees12/1 -> pw demand dead zone/1
  Product/1 -> Switch/3
  FCS_long_qVt_alim_pw/1 -> Radians to Degrees12/1
  pw demand dead zone/1 -> Product/2, Logical Operator5/1
  Logical Operator5/1 -> Logical Operator3/3

== system admire_fcs_lin/Control system1/FCS_long/FCS_long_qVt/FCS_long_qVt_fcslong ==
  note: Level V
  note: S-function
  FCS_long_qVt_fcslong_Altitude : Inport  Port=1  PortWidth=-1  SampleTime=-1  DataType=auto
      settings: SignalType=auto
  FCS_long_qVt_fcslong_Mach : Inport  Port=2  PortWidth=-1  SampleTime=-1  DataType=auto
      settings: SignalType=auto
  S-Function1 : S-Function  FunctionName=fcslongitudinal  PortCounts=[]  SFunctionModules=''
  FCS_long_qVt_fcslong_Kvt : Outport  Port=1
  FCS_long_qVt_fcslong_Kalfa : Outport  Port=2
  FCS_long_qVt_fcslong_Kq : Outport  Port=3
  FCS_long_qVt_fcslong_KI : Outport  Port=4
  FCS_long_qVt_fcslong_KP : Outport  Port=5
  wires:
  FCS_long_qVt_fcslong_Mach/1 -> S-Function1/2
  FCS_long_qVt_fcslong_Altitude/1 -> S-Function1/1
  S-Function1/1 -> FCS_long_qVt_fcslong_Kalfa/1
  S-Function1/2 -> FCS_long_qVt_fcslong_KI/1
  S-Function1/3 -> FCS_long_qVt_fcslong_KP/1
  S-Function1/4 -> FCS_long_qVt_fcslong_Kq/1
  S-Function1/5 -> FCS_long_qVt_fcslong_Kvt/1

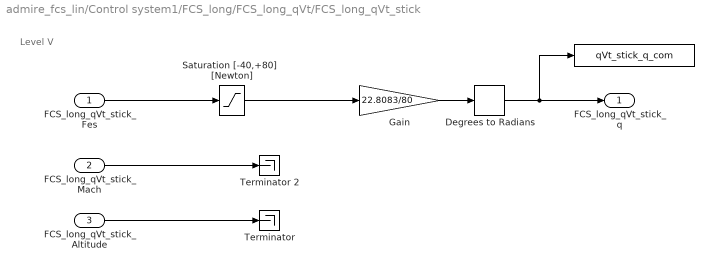
== system admire_fcs_lin/Control system1/FCS_long/FCS_long_qVt/FCS_long_qVt_stick ==
  note: Level V
  "FCS_long_qVt_stick_Fes " : Inport  Port=1  PortWidth=-1  SampleTime=-1  DataType=auto
      settings: SignalType=auto
  "FCS_long_qVt_stick_Mach " : Inport  Port=2  PortWidth=-1  SampleTime=-1  DataType=auto
      settings: SignalType=auto
  "FCS_long_qVt_stick_Altitude " : Inport  Port=3  PortWidth=-1  SampleTime=-1  DataType=auto
      settings: SignalType=auto
  " " : ToWorkspace  VariableName=qVt_stick_q_com  SampleTime=-1  SaveFormat=Matrix
  Degrees to Radians : simulink_extras/Transformations/Degrees to Radians
  Gain : Gain  Gain=22.8083/80  SaturateOnIntegerOverflow=on
  Saturation [-40,+80]   [Newton] : Saturate  UpperLimit=80  LowerLimit=-40
  Terminator : Terminator
  Terminator 2 : Terminator
  "FCS_long_qVt_stick_q " : Outport  Port=1
  wires:
  Gain/1 -> Degrees to Radians/1
  "FCS_long_qVt_stick_Altitude "/1 -> Terminator/1
  "FCS_long_qVt_stick_Fes "/1 -> Saturation [-40,+80]   [Newton]/1
  "FCS_long_qVt_stick_Mach "/1 -> Terminator 2/1
  Degrees to Radians/1 -> "FCS_long_qVt_stick_q "/1, " "/1
  Saturation [-40,+80]   [Newton]/1 -> Gain/1

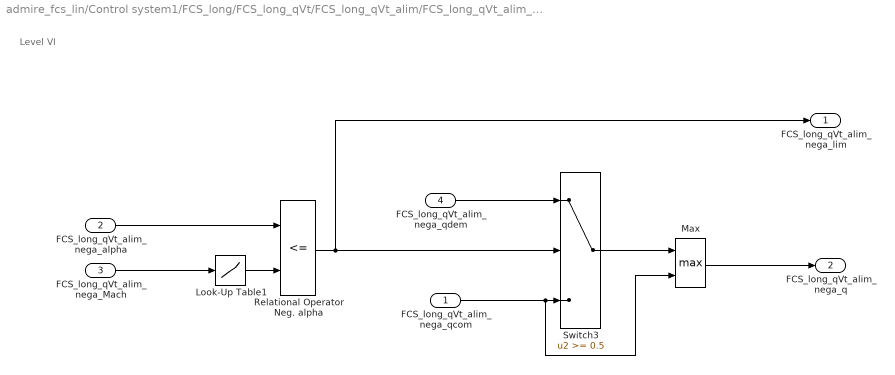
== system admire_fcs_lin/Control system1/FCS_long/FCS_long_qVt/FCS_long_qVt_alim/FCS_long_qVt_alim_nega ==
  note: Level VI
  "FCS_long_qVt_alim_nega_qcom " : Inport  Port=1  PortWidth=-1  SampleTime=-1  DataType=auto
      settings: SignalType=auto
  "FCS_long_qVt_alim_nega_alpha " : Inport  Port=2  PortWidth=-1  SampleTime=-1  DataType=auto
      settings: SignalType=auto
  "FCS_long_qVt_alim_nega_Mach " : Inport  Port=3  PortWidth=-1  SampleTime=-1  DataType=auto
      settings: SignalType=auto
  "FCS_long_qVt_alim_nega_qdem " : Inport  Port=4  PortWidth=-1  SampleTime=-1  DataType=auto
      settings: SignalType=auto
  Look-Up Table1 : Lookup  InputValues=[0 1 1 2.5]  OutputValues=[-8 -8 -3 -3]
  Max : MinMax  Function=max  Inputs=2
  Relational Operator Neg. alpha : RelationalOperator  Operator=<=
  Switch3 : Switch  Threshold=0.5
  FCS_long_qVt_alim_nega_lim : Outport  Port=1
  "FCS_long_qVt_alim_nega_q " : Outport  Port=2
  wires:
  "FCS_long_qVt_alim_nega_Mach "/1 -> Look-Up Table1/1
  Look-Up Table1/1 -> Relational Operator Neg. alpha/2
  "FCS_long_qVt_alim_nega_alpha "/1 -> Relational Operator Neg. alpha/1
  Max/1 -> "FCS_long_qVt_alim_nega_q "/1
  "FCS_long_qVt_alim_nega_qdem "/1 -> Switch3/1
  Relational Operator Neg. alpha/1 -> Switch3/2, FCS_long_qVt_alim_nega_lim/1
  Switch3/1 -> Max/1
  "FCS_long_qVt_alim_nega_qcom "/1 -> Switch3/3, Max/2

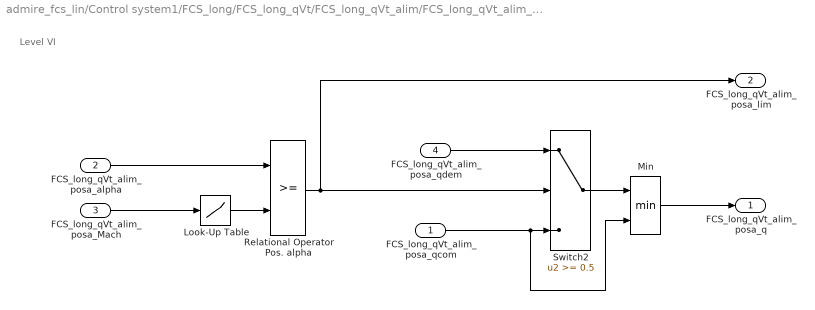
== system admire_fcs_lin/Control system1/FCS_long/FCS_long_qVt/FCS_long_qVt_alim/FCS_long_qVt_alim_posa ==
  note: Level VI
  "FCS_long_qVt_alim_posa_qcom " : Inport  Port=1  PortWidth=-1  SampleTime=-1  DataType=auto
      settings: SignalType=auto
  "FCS_long_qVt_alim_posa_alpha " : Inport  Port=2  PortWidth=-1  SampleTime=-1  DataType=auto
      settings: SignalType=auto
  "FCS_long_qVt_alim_posa_Mach " : Inport  Port=3  PortWidth=-1  SampleTime=-1  DataType=auto
      settings: SignalType=auto
  "FCS_long_qVt_alim_posa_qdem " : Inport  Port=4  PortWidth=-1  SampleTime=-1  DataType=auto
      settings: SignalType=auto
  Look-Up Table : Lookup  InputValues=[0 0.8 0.8 1 1 1.3 1.3 2.5 ]  OutputValues=[28 28 23 23 18 18 13 13 ]
  Min : MinMax  Function=min  Inputs=2
  Relational Operator Pos. alpha : RelationalOperator  Operator=>=
  Switch2 : Switch  Threshold=0.5
  FCS_long_qVt_alim_posa_q : Outport  Port=1
  FCS_long_qVt_alim_posa_lim : Outport  Port=2
  wires:
  "FCS_long_qVt_alim_posa_alpha "/1 -> Relational Operator Pos. alpha/1
  "FCS_long_qVt_alim_posa_Mach "/1 -> Look-Up Table/1
  Look-Up Table/1 -> Relational Operator Pos. alpha/2
  Relational Operator Pos. alpha/1 -> Switch2/2, FCS_long_qVt_alim_posa_lim/1
  "FCS_long_qVt_alim_posa_qdem "/1 -> Switch2/1
  Min/1 -> FCS_long_qVt_alim_posa_q/1
  Switch2/1 -> Min/1
  "FCS_long_qVt_alim_posa_qcom "/1 -> Switch2/3, Min/2
